simulink model "tianpeng"  (R2019a)
settings: Solver=VariableStepAuto  StartTime=0.0  StopTime=30  RelTol=1e-3
settings Model: Creator=91516  LastModifiedBy=91516

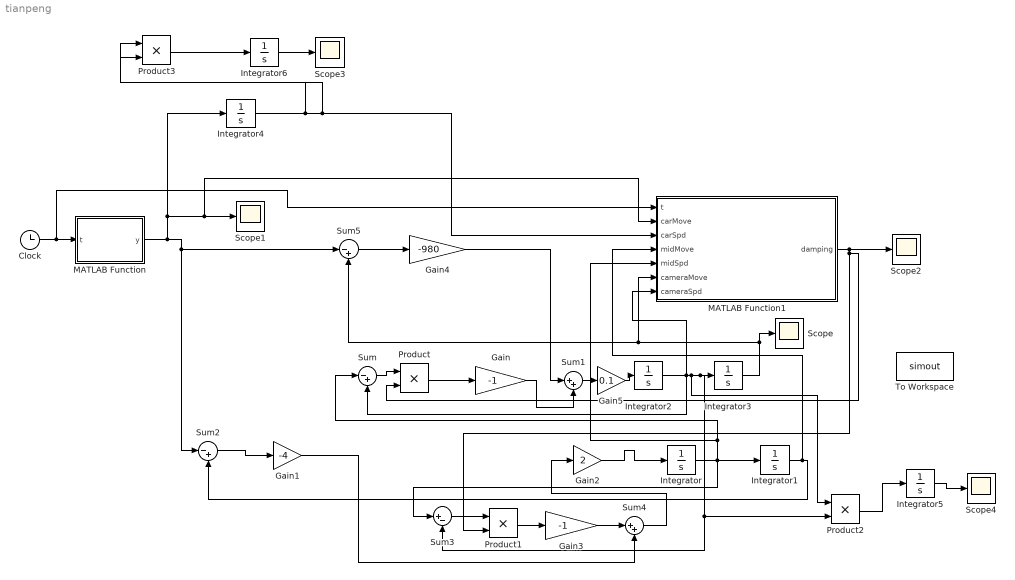
== system tianpeng ==
  Clock : Clock
      settings: Decimation=1000
  Gain : Gain  Gain=-1
  Gain1 : Gain  Gain=-4
  Gain2 : Gain  Gain=2
  Gain3 : Gain  Gain=-1
  Gain4 : Gain  Gain=-980
  Gain5 : Gain  Gain=0.1
  Integrator{,1..6} (7 alike) : Integrator
  MATLAB Function : MATLAB Function  TreatAsAtomicUnit=on
  MATLAB Function1 : MATLAB Function  TreatAsAtomicUnit=on
  Product{,1..3} (4 alike) : Product
  Scope{,1..4} (5 alike) : Scope
  Sum : Sum  Inputs=|-+
  Sum1 : Sum  Inputs=|++
  Sum2 : Sum  Inputs=|-+
  Sum3 : Sum  Inputs=|+-
  Sum4 : Sum  Inputs=|++
  Sum5 : Sum  Inputs=|-+
  To Workspace : ToWorkspace  VariableName=simout  SaveFormat=Timeseries  SampleTime=-1
  wires:
  Clock/1 -> MATLAB Function1/1(t), MATLAB Function/1(t)
  MATLAB Function/1(y) -> Integrator4/1, MATLAB Function1/2(carMove), Scope1/1, Sum5/1, Sum2/1
  Sum/1 -> Product/1
  Product/1 -> Gain/1
  Sum2/1 -> Gain1/1
  Gain2/1 -> Integrator/1
  Integrator1/1 -> MATLAB Function1/4(midMove), Sum2/2
  Sum3/1 -> Product1/1
  Product1/1 -> Gain3/1
  Gain3/1 -> Sum4/1
  Gain1/1 -> Sum4/2
  Integrator/1 -> MATLAB Function1/5(midSpd), Sum/1, Integrator1/1, Sum3/1
  Sum4/1 -> Gain2/1
  Sum5/1 -> Gain4/1
  Gain4/1 -> Sum1/1
  Gain/1 -> Sum1/2
  Integrator2/1 -> Product2/2, Sum3/2, Integrator3/1, Product2/1, MATLAB Function1/7(cameraSpd), Sum/2
  Integrator3/1 -> MATLAB Function1/6(cameraMove), Sum5/2, Scope/1
  MATLAB Function1/1(damping) -> Scope2/1, Product1/2, Product/2
  Sum1/1 -> Gain5/1
  Gain5/1 -> Integrator2/1
  Integrator4/1 -> Product3/1, Product3/2, MATLAB Function1/3(carSpd)
  Product3/1 -> Integrator6/1
  Integrator6/1 -> Scope3/1
  Product2/1 -> Integrator5/1
  Integrator5/1 -> Scope4/1

== matlab function tianpeng/MATLAB Function1 ==
  data: t input; carMove input; damping output; carSpd input; midMove input; midSpd input; cameraMove input; cameraSpd input
function damping = tianpengDamping(t,carMove,carSpd,midMove,midSpd,cameraMove,cameraSpd)
    speed=3;
    roadMove=5*sin(t*speed/20)+0.5*sin(t*speed/4)+0.3*sin(t*speed*6)+0.02*sin(t*speed*30)+0.3*sin(t*speed*60);
    idealforce=-25*(cameraMove-roadMove);
    if(cameraSpd-cameraMove==0)
        spdDif=0.001;
    else
        spdDif=cameraSpd-cameraMove;
    end
    idealDamping=-(idealforce+980*(cameraMove-midMove))/spdDif;
    if(idealDamping>2400)
        idealDamping=2400;
    else
        if(idealDamping<600)
            idealDamping=600;
        end
    end
    damping=idealDamping;
    %damping=100;
end

== matlab function tianpeng/MATLAB Function ==
  data: t input; y output
function y = sinRandomRoad(t)
    speed=3;
    y=5*sin(t*speed/20)+0.5*sin(t*speed/4)+0.3*sin(t*speed*6)+0.02*sin(t*speed*30)+0.3*sin(t*speed*60);
end
